simulink model "LQR_sfunc_2016a"  (R2015a)
settings: Solver=ode3  StartTime=0.0  StopTime=30  FixedStep=8e-5  RelTol=1e-3
values from neighbouring files (symbols this model uses):
  a = 1.035    [initParams.m]    (also in teste.m = 1.1; vsfmodel.m = block.DialogPrm(6).Data)
  b = 1.655    [initParams.m]    (also in teste.m = 1.3; vsfmodel.m = block.DialogPrm(7).Data)
  d = block.DialogPrm(10).Data    [vsfmodel.m]
  LQRopt = lqrd(A,B,Q,R,8e-5)    [initParams.m]    (also in teste.m)
  MFA = [ 1.6  ,-34 , 1250 ,  23200 , 12.8 , 0    , -0.0053, 0.1925 ]    [initParams.m]    (also in teste.m = [ 1.6  ,-34 , 1250 ,  2320  , 12.8 ,     0 , -0.0053 , 0.192; vsfmodel.m = block.DialogPrm(1).Data)
  MFB = [ 1.55 ,0   , 1000 ,   60  , 300  , 0.17 , 0      , 0      ,0.2 ]    [initParams.m]    (also in teste.m; vsfmodel.m = block.DialogPrm(2).Data)
  z = block.DialogPrm(3).Data    [vsfmodel.m]
  zf0 = m*g*b/(2*l)    (= 5139.13184015)    [initParams.m]    (also in teste.m = 2841.88544792; vsfmodel.m = block.DialogPrm(4).Data)
  zr0 = m*g*a/(2*l)    (= 3213.89815985)    [initParams.m]    (also in teste.m = 2404.67230208; vsfmodel.m = block.DialogPrm(5).Data)
undefined symbols (not defined in the file or in its folder): t2
settings Model: Creator=zoero  LastModifiedBy=zoero
settings SolverCC: PositivePriorityOrder=on

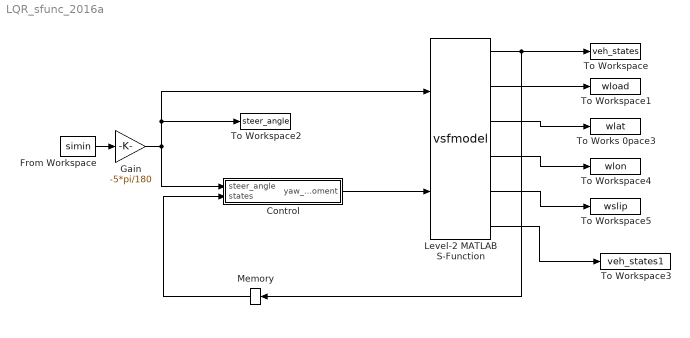
== system LQR_sfunc_2016a ==
  "Control " : Subsystem  TreatAsAtomicUnit=on
  From Workspace : FromWorkspace  VariableName=simin  SampleTime=0
  Gain : Gain  Gain=-5*pi/180
  Level-2 MATLAB S-Function : M-S-Function  FunctionName=vsfmodel  Parameters=MFA,MFB,z,zf0,zr0,a,b,t2,d,60/3.6
  Memory : Memory  X0=[0,60/3.6,0,0,0]
  To Works 0pace3 : ToWorkspace  VariableName=wlat  SaveFormat=Timeseries  SampleTime=-1
  To Workspace : ToWorkspace  VariableName=veh_states  SaveFormat=Timeseries  SampleTime=-1
  To Workspace1 : ToWorkspace  VariableName=wload  SaveFormat=Timeseries  SampleTime=-1
  To Workspace2 : ToWorkspace  VariableName=steer_angle  SaveFormat=Timeseries  SampleTime=-1
  To Workspace3 : ToWorkspace  VariableName=veh_states1  SaveFormat=Timeseries  SampleTime=-1
  To Workspace4 : ToWorkspace  VariableName=wlon  SaveFormat=Timeseries  SampleTime=-1
  To Workspace5 : ToWorkspace  VariableName=wslip  SaveFormat=Timeseries  SampleTime=-1
  wires:
  From Workspace/1 -> Gain/1
  Gain/1 -> Level-2 MATLAB S-Function/1, To Workspace2/1, "Control "/1(steer_angle)
  "Control "/1(yaw_moment) -> Level-2 MATLAB S-Function/2
  Memory/1 -> "Control "/2(states)
  Level-2 MATLAB S-Function/1 -> Memory/1, To Workspace/1
  Level-2 MATLAB S-Function/2 -> To Workspace1/1
  Level-2 MATLAB S-Function/3 -> To Works 0pace3/1
  Level-2 MATLAB S-Function/4 -> To Workspace4/1
  Level-2 MATLAB S-Function/5 -> To Workspace5/1
  Level-2 MATLAB S-Function/6 -> To Workspace3/1

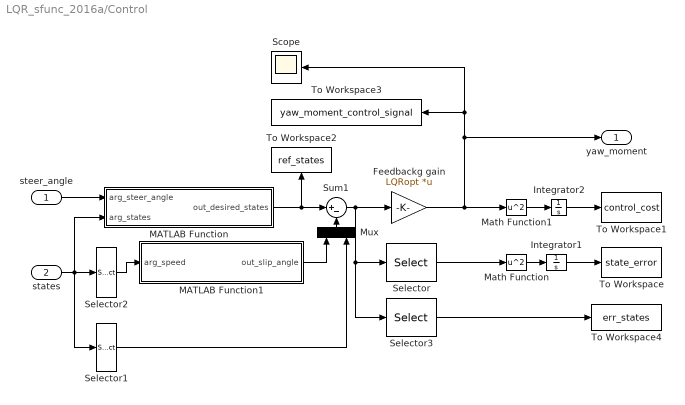
== system LQR_sfunc_2016a/Control  ==
  steer_angle : Inport
  states : Inport  Port=2
  Feedbackg gain : Gain  Gain=LQRopt  Multiplication=Matrix(K*u)
  Integrator1 : Integrator
  Integrator2 : Integrator
  MATLAB Function : MATLAB Function  TreatAsAtomicUnit=on
  MATLAB Function1 : MATLAB Function  TreatAsAtomicUnit=on
  Math Function : Math  Operator=square  SaturateOnIntegerOverflow=on
  Math Function1 : Math  Operator=square  SaturateOnIntegerOverflow=on
  Mux : Mux  Inputs=2
  Scope : Scope
      settings: YMin=-1.00000  YMax=1.00000
  Selector : Selector  InputPortWidth=4  Indices=[1 2]
  Selector1 : Selector  InputPortWidth=5  Indices=[3,4,5]
  Selector2 : Selector  InputPortWidth=5  Indices=[1,2]
  Selector3 : Selector  InputPortWidth=4  Indices=[1 2]
  Sum1 : Sum  Inputs=|+-
  To Workspace : ToWorkspace  VariableName=state_error  SaveFormat=Timeseries  SampleTime=-1
      settings: MaxDataPoints=1
  To Workspace1 : ToWorkspace  VariableName=control_cost  SaveFormat=Timeseries  SampleTime=-1
      settings: MaxDataPoints=1
  To Workspace2 : ToWorkspace  VariableName=ref_states  SaveFormat=Timeseries  SampleTime=-1
      settings: MaxDataPoints=Inf
  To Workspace3 : ToWorkspace  VariableName=yaw_moment_control_signal  SaveFormat=Timeseries  SampleTime=-1
      settings: MaxDataPoints=Inf
  To Workspace4 : ToWorkspace  VariableName=err_states  SaveFormat=Timeseries  SampleTime=-1
      settings: MaxDataPoints=Inf
  yaw_moment : Outport
  wires:
  Feedbackg gain/1 -> To Workspace3/1, Scope/1, yaw_moment/1, Math Function1/1
  steer_angle/1 -> MATLAB Function/1(arg_steer_angle)
  Math Function/1 -> Integrator1/1
  Integrator1/1 -> To Workspace/1
  Math Function1/1 -> Integrator2/1
  Integrator2/1 -> To Workspace1/1
  Selector/1 -> Math Function/1
  MATLAB Function/1(out_desired_states) -> Sum1/1, To Workspace2/1
  states/1 -> MATLAB Function/2(arg_states), Selector1/1, Selector2/1
  MATLAB Function1/1(out_slip_angle) -> Mux/1
  Selector2/1 -> MATLAB Function1/1(arg_speed)
  Mux/1 -> Sum1/2
  Selector1/1 -> Mux/2
  Sum1/1 -> Selector3/1, Selector/1, Feedbackg gain/1
  Selector3/1 -> To Workspace4/1

== matlab function LQR_sfunc_2016a/Control /MATLAB Function1 ==
  data: arg_speed input; out_slip_angle output
function out_slip_angle = slipangle(arg_speed)

out_slip_angle = atan2(arg_speed(1),arg_speed(2));

== matlab function LQR_sfunc_2016a/Control /MATLAB Function ==
  data: arg_steer_angle input; out_desired_states output; arg_states input
function  out_desired_states  = desired_states( arg_steer_angle, arg_states )

persistent mu_g;
persistent Ku;
persistent l;

if isempty(Ku)
    modelParams = coder.load( 'modelParam.mat' );
    mu_g = modelParams.friction_coefficient*modelParams.g;
    l = modelParams.l;
    Ku = modelParams.Ku;
end

long_speed = arg_states(2);
lat_speed = arg_states(1);
speed = sqrt(long_speed*long_speed + lat_speed*lat_speed);
aux = l*(1 + Ku*speed*speed);
desired_yaw_rate =  speed*arg_steer_angle/aux;
desired_yaw_rate = min([abs(desired_yaw_rate), abs(mu_g/speed)])*sign(arg_steer_angle);

desired_slip = atan2(arg_states(1),arg_states(2));
if abs(desired_slip) > (10*pi/180) 
    desired_slip = 10*pi/180*sign(desired_slip);
end

out_desired_states = [desired_slip; desired_yaw_rate; 0; 0 ];

end
